simulink model "sampleModel1786_1"  (R2023a)
settings: Solver=VariableStepAuto  StartTime=0.0  StopTime=10.0  RelTol=1e-3
libraries: hdlsllib x2, simulink x2
settings Model: Creator=user1  LastModifiedBy=user1

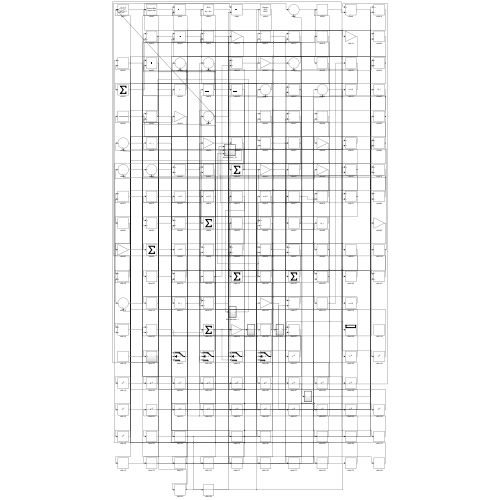
[thumbnail: Simulink's stored preview of the top-level diagram]
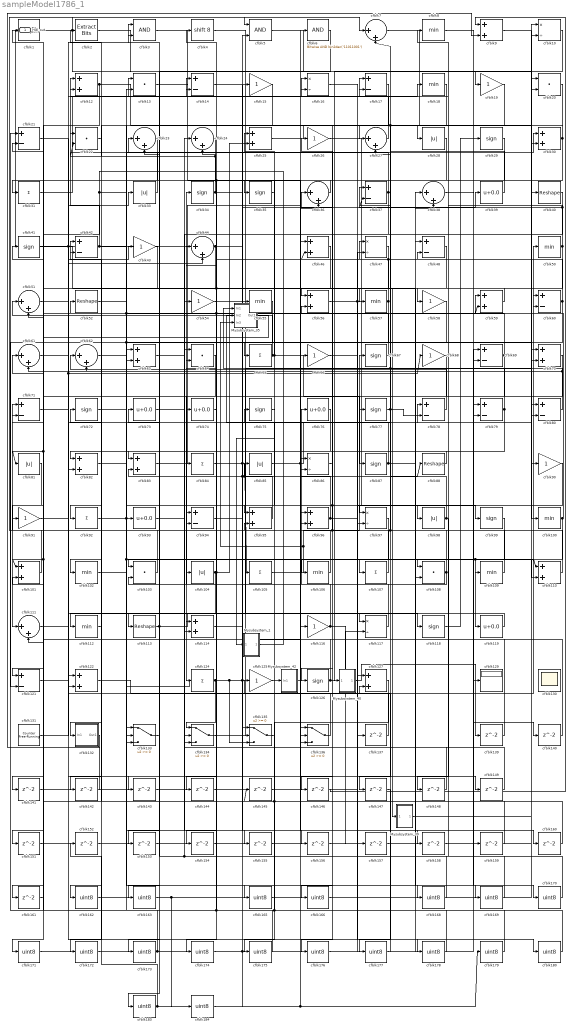
== system sampleModel1786_1 ==
  Mysubsystem_1 : Subsystem  TreatAsAtomicUnit=on  RTWFcnName=Mysubsystem_1
      settings: RTWFcnNameOpts=User specified  RTWFileNameOpts=Use function name
  Mysubsystem_35 : Subsystem  TreatAsAtomicUnit=on  RTWFcnName=Mysubsystem_35
      settings: RTWFcnNameOpts=User specified  RTWFileNameOpts=Use function name
  Mysubsystem_39 : Subsystem  TreatAsAtomicUnit=on  RTWFcnName=Mysubsystem_39
      settings: RTWFcnNameOpts=User specified  RTWFileNameOpts=Use function name
  Mysubsystem_40 : Subsystem  TreatAsAtomicUnit=on  RTWFcnName=Mysubsystem_40
      settings: RTWFcnNameOpts=User specified  RTWFileNameOpts=Use function name
  Mysubsystem_42 : Subsystem  TreatAsAtomicUnit=on  RTWFcnName=Mysubsystem_42
      settings: RTWFcnNameOpts=User specified  RTWFileNameOpts=Use function name
  cfblk1 : hdlsllib/Logic and Bit Operations/Detect Rise Nonnegative  vinit=0  OutDataTypeStr=uint8
  cfblk{10,16,47,86,97,117} (6 alike) : Product  Inputs=*/  OutDataTypeStr=uint8  RndMeth=Zero  SaturateOnIntegerOverflow=on
  cfblk{8,18,50,55,57,100,102,106,109,112} (10 alike) : MinMax  OutDataTypeStr=uint8
  cfblk{9,12,25,30,46,56,59,63,70,82..83,95..96,101,110,114,122,127} (18 alike) : Sum  OutDataTypeStr=uint8
  cfblk{13,20,22,64,103,108} (6 alike) : DotProduct  OutDataTypeStr=uint8
  cfblk{28,33,81,85,98,104} (6 alike) : Abs  OutDataTypeStr=uint8  SaturateOnIntegerOverflow=off
  cfblk{31,65,84,92,105,107,124} (7 alike) : Sum  Inputs=+  OutDataTypeStr=uint8
  cfblk{7,23..24,27,36,38,44,51,61..62,111} (11 alike) : Sum  Inputs=|++  OutDataTypeStr=uint8
  cfblk{40,52,88,113} (4 alike) : Reshape
  cfblk{15,19,26,43,54,58,66,68,90..91,116,125} (12 alike) : Gain  OutDataTypeStr=uint8
  cfblk{29,34..35,41,67,72,75,77,87,99,118,126} (12 alike) : Signum
  cfblk{39,73..74,76,93,119} (6 alike) : Bias  Bias=0.0  SaturateOnIntegerOverflow=off
  cfblk{14,17,21,37,42,48,60,69,71,78..80,94,121} (14 alike) : Sum  Inputs=+-  OutDataTypeStr=uint8
  cfblk129 : Display
  cfblk130 : Scope
      settings: Floating=on
  cfblk131 : hdlsllib/Sources/Counter Free-Running  NumBits=16  tsamp=-1
  cfblk132 : Subsystem
      settings: LibrarySourceBlock=|
      | hdlsllib/Ports &
      | Subsystems/Subsystem
  cfblk{133..136} (4 alike) : Switch  OutDataTypeStr=uint8  SaturateOnIntegerOverflow=off  InputSameDT=off
  cfblk{137,139..149,151..161} (23 alike) : Delay  SampleTime=1
  cfblk{162..163,165..166,168..180,183..184} (19 alike) : DataTypeConversion  OutDataTypeStr=uint8  SaturateOnIntegerOverflow=off  RndMeth=Floor
  cfblk2 : simulink/Logic and Bit Operations/Extract Bits  bitsToExtract=Upper half  numBits=8  bitIdxRange=[0 7]  outScalingMode=Preserve fixed-point scaling
      settings: LibrarySourceBlock=|
      | hdlsllib/Logic and Bit
      | Operations/Extract Bits
  cfblk3 : Logic  AllPortsSameDT=off  OutDataTypeStr=boolean
  cfblk4 : ArithShift  BitShiftNumber=8
  cfblk5 : Logic  AllPortsSameDT=off  OutDataTypeStr=boolean
  cfblk6 : simulink/Logic and Bit Operations/Bitwise Operator  logicop=AND  UseBitMask=on  BitMask=bin2dec('11011001')  BitMaskRealWorld=Stored Integer
      settings: LibrarySourceBlock=|
      | hdlsllib/Logic and Bit
      | Operations/Bitwise
      | Operator
  Hdl_out : Outport  OutDataTypeStr=uint8
  wires:
  cfblk4/1 -> cfblk118/1
  cfblk36/1 -> cfblk35/1
  cfblk127/1 -> cfblk175/1
  cfblk6/1 -> cfblk163/1
  cfblk25/1 -> cfblk28/1
  cfblk88/1 -> cfblk82/1
  cfblk118/1 -> cfblk29/1
  cfblk119/1 -> cfblk113/1
  cfblk116/1 -> cfblk34/1, cfblk157/1
  cfblk122/1 -> cfblk50/1
  cfblk87/1 -> Mysubsystem_35/2(In2), cfblk169/1
  cfblk29/1 -> cfblk65/1
  cfblk56/1 -> cfblk99/1, cfblk110/2
  cfblk117/1 -> cfblk76/1
  cfblk101/1 -> cfblk5/1
  cfblk109/1 -> cfblk71/1
  cfblk80/1 -> cfblk36/1
  cfblk23/1 -> cfblk31/1
  cfblk113/1 -> cfblk117/1, cfblk153/1
  cfblk7/1 -> cfblk80/1
  cfblk133/1 -> cfblk73/1
  cfblk100/1 -> cfblk108/1, cfblk60/1
  cfblk17/1 -> cfblk112/1
  cfblk15/1 -> cfblk183/1
  cfblk81/1 -> cfblk111/1
  cfblk103/1 -> cfblk72/1
  cfblk124/1 -> cfblk40/1, cfblk60/2, cfblk135/3, cfblk134/1
  cfblk2/1 -> cfblk19/1
  cfblk43/1 -> cfblk111/2
  cfblk92/1 -> cfblk74/1, cfblk158/1
  cfblk64/1 -> cfblk124/1
  cfblk18/1 -> cfblk63/2
  cfblk27/1 -> cfblk16/1
  cfblk24/1 -> cfblk82/2, cfblk22/2
  cfblk3/1 -> cfblk96/1
  cfblk84/1 -> cfblk105/1, cfblk56/2
  cfblk33/1 -> cfblk12/1
  cfblk35/1 -> cfblk95/1
  cfblk62/1 -> cfblk133/1, cfblk110/1
  cfblk67/1 -> cfblk41/1, cfblk4/1
  cfblk54/1 -> cfblk39/1
  cfblk21/1 -> cfblk178/1
  cfblk107/1 -> cfblk23/1, cfblk26/1
  cfblk105/1 -> Mysubsystem_35/3(In3), cfblk67/1
  cfblk104/1 -> cfblk64/2, cfblk25/2, cfblk132/1(In1)
  cfblk22/1 -> cfblk102/1
  cfblk12/1 -> cfblk129/1, cfblk161/1
  cfblk26/1 -> cfblk100/1
  cfblk19/1 -> cfblk126/1
  cfblk9/1 -> cfblk90/1
  cfblk58/1 -> cfblk92/1
  cfblk5/1 -> cfblk79/2
  cfblk111/1 -> cfblk78/1
  cfblk83/1 -> cfblk17/1
  cfblk126/1 -> cfblk52/1, cfblk117/2
  cfblk50/1 -> cfblk12/2, cfblk37/2, cfblk57/1
  cfblk13/1 -> cfblk16/2
  cfblk31/1 -> cfblk14/1
  cfblk37/1 -> cfblk97/1, cfblk3/2, cfblk134/3
  cfblk52/1 -> cfblk93/1, cfblk106/1
  cfblk79/1 -> Mysubsystem_35/1(In1), cfblk7/2, cfblk142/1
  cfblk65/1 -> cfblk87/1, cfblk25/1, cfblk51/1
  cfblk47/1 -> cfblk84/1, cfblk172/1, cfblk46/2
  cfblk55/1 -> cfblk173/1
  cfblk99/1 -> cfblk119/1, cfblk154/1
  cfblk70/1 -> cfblk61/2, cfblk114/2
  cfblk134/1 -> cfblk66/1
  cfblk131/1 -> cfblk17/2, cfblk68/1
  cfblk34/1 -> cfblk56/1, cfblk2/1
  cfblk98/1 -> cfblk77/1, cfblk148/1
  cfblk14/1 -> cfblk109/1
  cfblk77/1 -> cfblk78/2, cfblk147/1
  cfblk85/1 -> cfblk20/1, cfblk160/1
  cfblk97/1 -> cfblk103/1
  cfblk57/1 -> cfblk13/1, cfblk136/3
  cfblk39/1 -> cfblk14/2
  cfblk78/1 -> cfblk62/1
  cfblk51/1 -> cfblk33/1
  cfblk28/1 -> cfblk121/1
  cfblk38/1 -> cfblk170/1
  cfblk90/1 -> cfblk133/3, cfblk146/1
  cfblk108/1 -> cfblk37/1, cfblk24/2, cfblk103/2
  cfblk112/1 -> cfblk62/2
  cfblk1/1 -> cfblk70/2, cfblk7/1
  cfblk44/1 -> cfblk122/2, cfblk18/1, Hdl_out/1
  cfblk68/1 -> cfblk94/1
  cfblk91/1 -> cfblk43/1
  cfblk132/1(Out1) -> cfblk9/2
  cfblk72/1 -> cfblk30/1, cfblk59/2
  cfblk41/1 -> cfblk108/2, cfblk3/1, cfblk114/1
  cfblk46/1 -> cfblk101/1, cfblk171/1
  cfblk20/1 -> cfblk107/1, cfblk135/2
  cfblk82/1 -> cfblk13/2
  cfblk66/1 -> cfblk98/1
  cfblk60/1 -> cfblk121/2, cfblk27/2
  cfblk42/1 -> cfblk69/2, cfblk168/1, cfblk22/1
  cfblk135/1 -> cfblk75/1
  cfblk61/1 -> cfblk44/2
  cfblk95/1 -> cfblk85/1, cfblk23/2
  cfblk69/1 -> cfblk81/1, cfblk91/1, cfblk47/1
  cfblk76/1 -> cfblk83/1
  cfblk114/1 -> cfblk59/1, cfblk88/1
  cfblk96/1 -> cfblk86/2, cfblk180/1
  cfblk73/1 -> cfblk24/1
  cfblk106/1 -> cfblk94/2
  cfblk125/1 -> cfblk86/1
  cfblk136/1 -> cfblk42/1
  cfblk63/1 -> cfblk54/1
  cfblk59/1 -> cfblk58/1
  cfblk110/1 -> cfblk8/1
  cfblk30/1 -> cfblk144/1, cfblk162/1, cfblk27/1
  cfblk16/1 -> cfblk137/1
  cfblk137/1 -> cfblk122/1
  cfblk139/1 -> cfblk44/1
  cfblk8/1 -> cfblk140/1
  cfblk140/1 -> cfblk1/1
  cfblk141/1 -> cfblk5/2
  cfblk142/1 -> cfblk101/2
  cfblk71/1 -> cfblk143/1
  cfblk143/1 -> cfblk136/1
  cfblk144/1 -> cfblk97/2
  cfblk145/1 -> cfblk95/2
  cfblk146/1 -> cfblk9/1
  cfblk148/1 -> cfblk134/2
  cfblk121/1 -> cfblk149/1
  cfblk149/1 -> cfblk46/1
  cfblk151/1 -> cfblk47/2
  cfblk152/1 -> cfblk30/2
  cfblk153/1 -> cfblk136/2
  cfblk154/1 -> cfblk36/2
  cfblk93/1 -> cfblk155/1
  cfblk155/1 -> cfblk80/2
  cfblk94/1 -> cfblk156/1
  cfblk156/1 -> cfblk20/2
  cfblk157/1 -> cfblk69/1
  cfblk158/1 -> cfblk79/1
  cfblk159/1 -> cfblk61/1
  cfblk160/1 -> cfblk42/2
  cfblk161/1 -> cfblk51/2
  cfblk162/1 -> cfblk6/1
  cfblk163/1 -> cfblk116/1, cfblk184/1
  cfblk102/1 -> cfblk165/1
  cfblk165/1 -> cfblk10/1
  cfblk40/1 -> cfblk166/1
  cfblk166/1 -> cfblk10/2
  cfblk168/1 -> cfblk48/1
  cfblk169/1 -> cfblk48/2
  cfblk170/1 -> cfblk83/2, cfblk64/1
  cfblk171/1 -> cfblk38/1
  cfblk172/1 -> cfblk38/2
  cfblk173/1 -> cfblk159/1, cfblk135/1, cfblk133/2
  cfblk74/1 -> cfblk174/1
  cfblk174/1 -> cfblk55/1
  cfblk175/1 -> cfblk104/1, cfblk63/1
  cfblk86/1 -> cfblk176/1
  cfblk176/1 -> cfblk127/1
  cfblk147/1 -> cfblk177/1
  cfblk177/1 -> cfblk127/2
  cfblk178/1 -> cfblk145/1, cfblk125/1, cfblk71/2
  cfblk179/1 -> cfblk21/1
  cfblk180/1 -> cfblk21/2
  cfblk183/1 -> cfblk179/1, cfblk96/2, cfblk152/1
  cfblk184/1 -> cfblk15/1
  Mysubsystem_1/1(Out1) -> Mysubsystem_42/1(In1), cfblk151/1
  cfblk75/1 -> Mysubsystem_1/1(In1)
  Mysubsystem_35/1(Out1) -> cfblk141/1
  cfblk48/1 -> Mysubsystem_39/1(In1)
  Mysubsystem_39/1(Out1) -> cfblk70/1
  cfblk10/1 -> Mysubsystem_40/1(In1)
  Mysubsystem_40/1(Out1) -> cfblk139/1

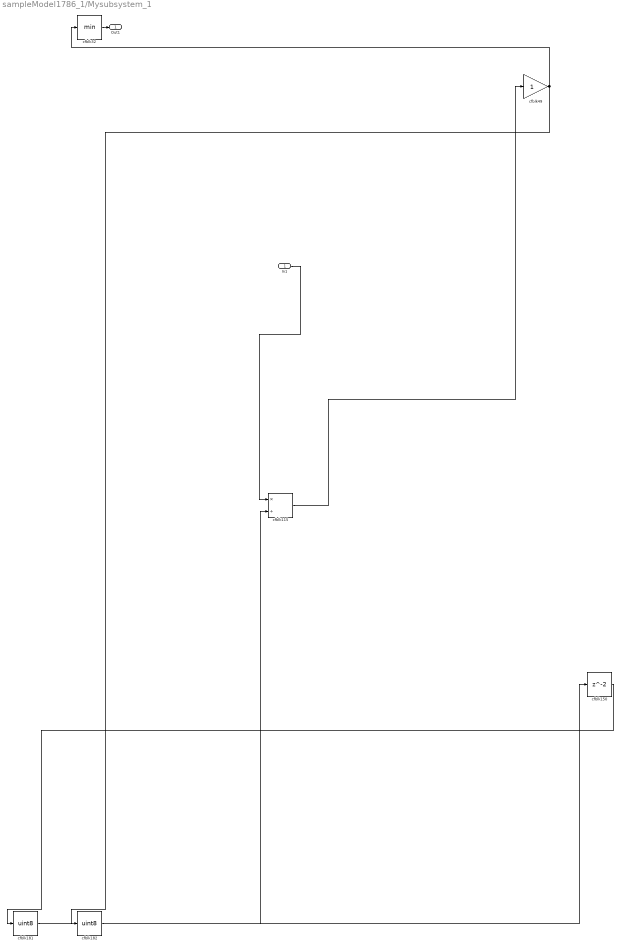
== system sampleModel1786_1/Mysubsystem_1 ==
  In1 : Inport
  cfblk115 : Product  Inputs=*/  RndMeth=Zero  SaturateOnIntegerOverflow=on
  cfblk150 : Delay  SampleTime=1
  cfblk181 : DataTypeConversion  OutDataTypeStr=uint8  SaturateOnIntegerOverflow=off  RndMeth=Floor
  cfblk182 : DataTypeConversion  OutDataTypeStr=uint8  SaturateOnIntegerOverflow=off  RndMeth=Floor
  cfblk32 : MinMax
  cfblk49 : Gain
  Out1 : Outport
  wires:
  cfblk181/1 -> cfblk115/2
  In1/1 -> cfblk115/1
  cfblk150/1 -> cfblk181/1
  cfblk115/1 -> cfblk49/1
  cfblk49/1 -> cfblk32/1, cfblk182/1
  cfblk182/1 -> cfblk150/1
  cfblk32/1 -> Out1/1

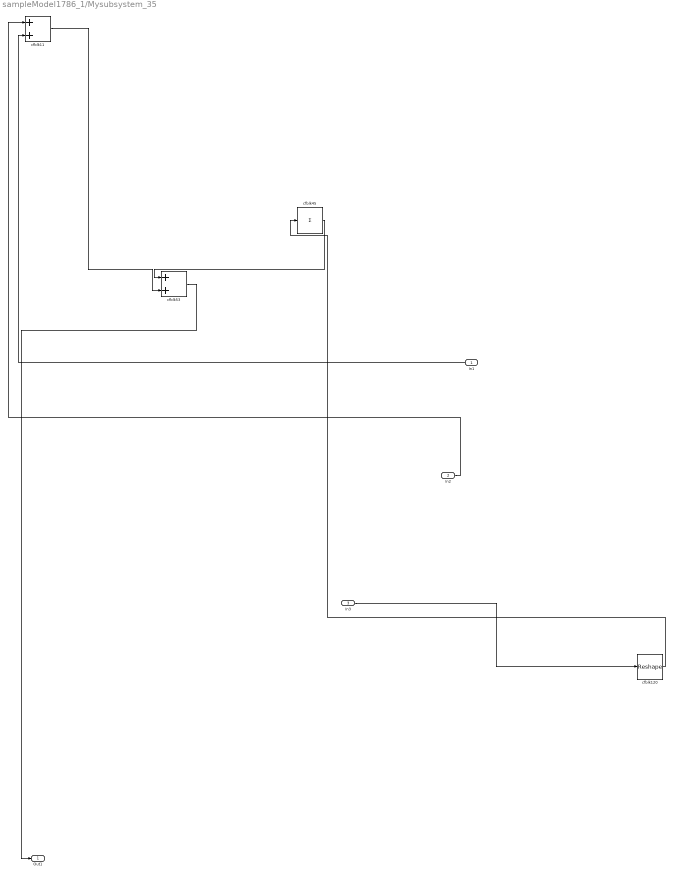
== system sampleModel1786_1/Mysubsystem_35 ==
  In1 : Inport
  In2 : Inport  Port=2
  In3 : Inport  Port=3
  cfblk11 : Sum
  cfblk120 : Reshape
  cfblk45 : Sum  Inputs=+
  cfblk53 : Sum
  Out1 : Outport
  wires:
  In3/1 -> cfblk120/1
  cfblk120/1 -> cfblk45/1
  cfblk53/1 -> Out1/1
  cfblk11/1 -> cfblk53/2
  cfblk45/1 -> cfblk53/1
  In1/1 -> cfblk11/2
  In2/1 -> cfblk11/1

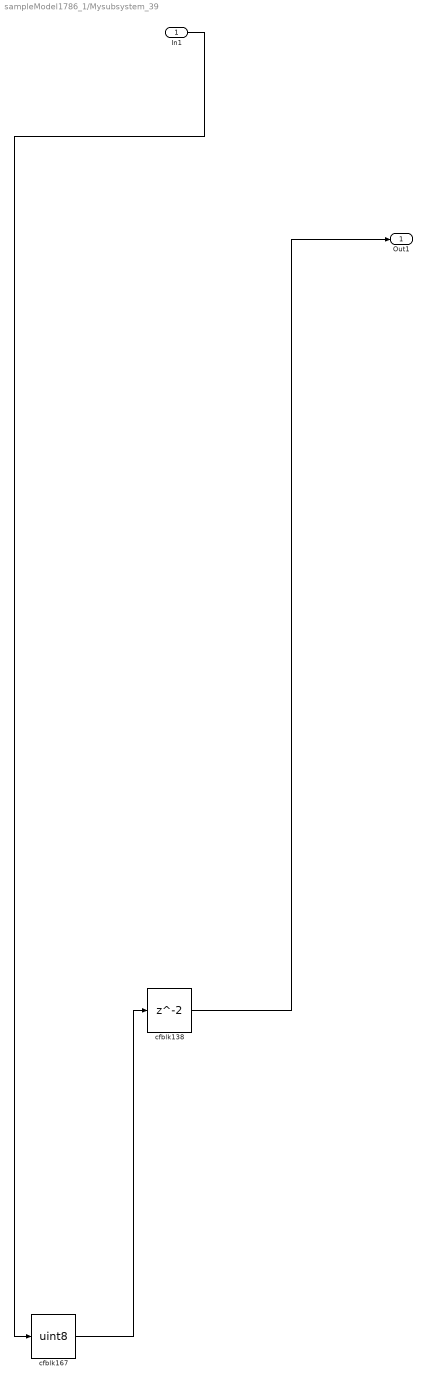
== system sampleModel1786_1/Mysubsystem_39 ==
  In1 : Inport
  cfblk138 : Delay  SampleTime=1
  cfblk167 : DataTypeConversion  OutDataTypeStr=uint8  SaturateOnIntegerOverflow=off  RndMeth=Floor
  Out1 : Outport
  wires:
  cfblk167/1 -> cfblk138/1
  cfblk138/1 -> Out1/1
  In1/1 -> cfblk167/1

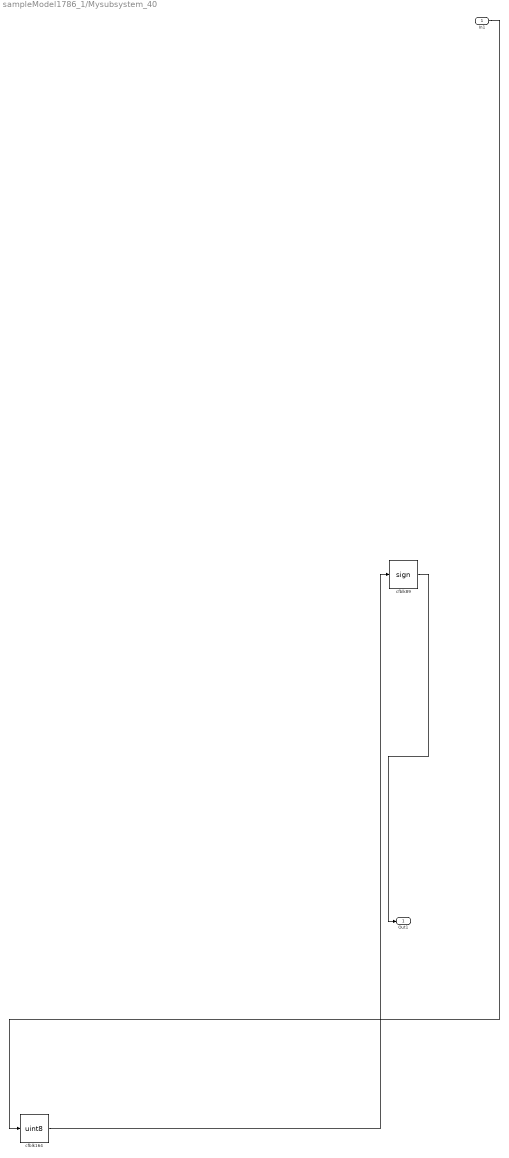
== system sampleModel1786_1/Mysubsystem_40 ==
  In1 : Inport
  cfblk164 : DataTypeConversion  OutDataTypeStr=uint8  SaturateOnIntegerOverflow=off  RndMeth=Floor
  cfblk89 : Signum
  Out1 : Outport
  wires:
  cfblk164/1 -> cfblk89/1
  cfblk89/1 -> Out1/1
  In1/1 -> cfblk164/1

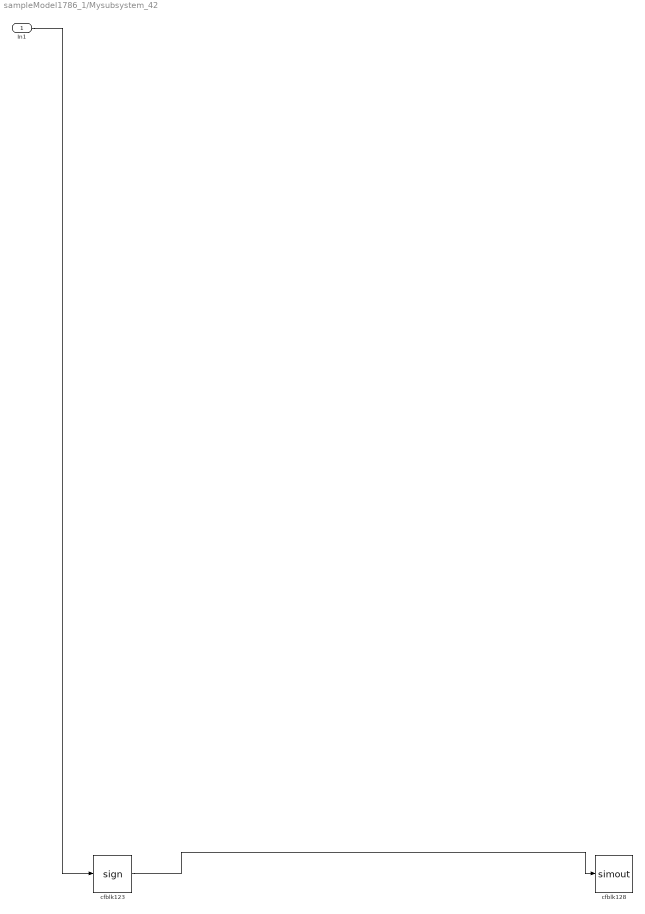
== system sampleModel1786_1/Mysubsystem_42 ==
  In1 : Inport
  cfblk123 : Signum
  cfblk128 : ToWorkspace  VariableName=simout  SaveFormat=Timeseries  SampleTime=-1
  wires:
  cfblk123/1 -> cfblk128/1
  In1/1 -> cfblk123/1

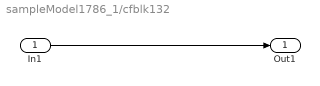
== system sampleModel1786_1/cfblk132 ==
  In1 : Inport
  Out1 : Outport
  wires:
  In1/1 -> Out1/1
